simulink model "transmittingModel"  (R2024b)
settings: Solver=VariableStepAuto  StartTime=0.0  StopTime=inf  RelTol=1e-3
undefined symbols (not defined in the file or in its folder): designMultirateFIR, Fs, ip, j, usb
libraries: plutoradiolib x3, dspmlti4 x1, dspvision x1
settings Model: Creator=jldis  LastModifiedBy=jldis

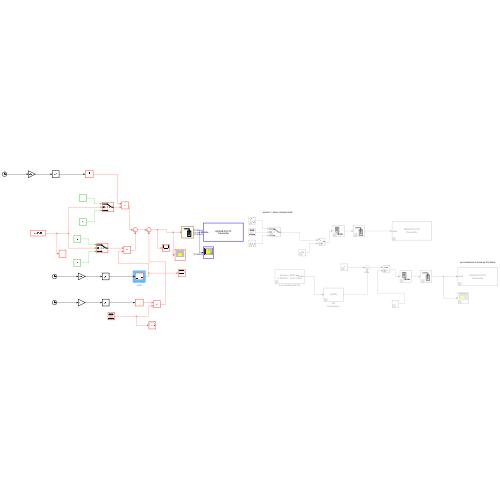
[thumbnail: Simulink's stored preview of the top-level diagram]
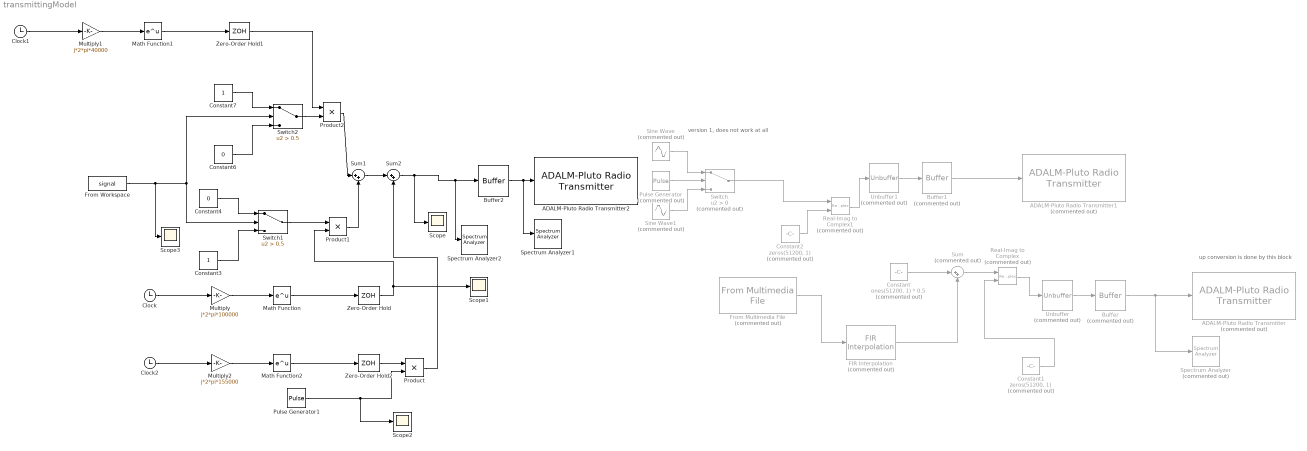
== system transmittingModel ==
  note: version 1, does not work at all
  note: up conversion is done by this block
  ADALM-Pluto Radio Transmitter : plutoradiolib/ADALM-Pluto Radio Transmitter  Commented=on  RadioID=usb:0  uri=ip:10.0.0.200  CenterFrequencySource=Dialog  CenterFrequency=915060000  GainSource=Dialog  Gain=-15  ChannelMapping=1  BasebandSampleRate=400000  UnderflowOutputPort=off  ShowAdvancedProperties=off  UseCustomFilter=off  filtPathRates=[737280000 11520000 3840000 1920000 960000 240000]  filtCoefficients=[-192 82 85 -215 228 -102 -110 290 -318 145 160 -426 471 -215 -238 633 -697 318 349 -923 1009 -457 -498 1309 -1423 640 693 -1812 1959 -876 -945 2458 -2647 1180 1268 -3290 3534 -1572 -1688 4375 -4698 2091 2247 -5836 6284 -2807 -3031 7918 -8588 3870 4225 -11182 12324 -5662 -6330 17255 -19735 9507 11312 -33568 43355 -25227 -42139 305542 305542 -42139 -25227 43355 -33568 11312 9507 -19735 17255 -6330 -5662 12324 -11182 4225 3870 -8588 7918 -3031 -2807 6284 -5836 2247 2091 -4698 4375 -1688 -1572 3534 -3290 1268 1180 -2647 2458 -945 -876 1959 -1812 693 640 -1423 1309 -498 -457 1009 -923 349 318 -697 633 -238 -215 471 -426 160 145 -318 290 -110 -102 228 -215 85 82 -192]  filtCoefficientSize=128  filtDecimInterpFactor=4  filtGain=-12  filtRFBandwidth=18000000  filterConfigStruct=struct()  DataSourceSelect=Input Port  DDSTone1Freq=5e3  DDSTone2Freq=10e3  DDSTone1Scale=0.5  DDSTone2Scale=0.25  DataTimeout=Inf  FrequencyCorrection=0  ENSMPinControlMode=None  BISTLoopbackMode=Disabled  BISTToneInject=Disabled  BISTSignalGen=PRBS  BISTToneFreq=Fs/32  BISTToneLevel=0
  ADALM-Pluto Radio Transmitter1 : plutoradiolib/ADALM-Pluto Radio Transmitter  Commented=on  RadioID=usb:0  uri=ip:10.0.0.200  CenterFrequencySource=Dialog  CenterFrequency=915060000  GainSource=Dialog  Gain=-15  ChannelMapping=1  BasebandSampleRate=400000  UnderflowOutputPort=off  ShowAdvancedProperties=off  UseCustomFilter=off  filtPathRates=[737280000 11520000 3840000 1920000 960000 240000]  filtCoefficients=[-192 82 85 -215 228 -102 -110 290 -318 145 160 -426 471 -215 -238 633 -697 318 349 -923 1009 -457 -498 1309 -1423 640 693 -1812 1959 -876 -945 2458 -2647 1180 1268 -3290 3534 -1572 -1688 4375 -4698 2091 2247 -5836 6284 -2807 -3031 7918 -8588 3870 4225 -11182 12324 -5662 -6330 17255 -19735 9507 11312 -33568 43355 -25227 -42139 305542 305542 -42139 -25227 43355 -33568 11312 9507 -19735 17255 -6330 -5662 12324 -11182 4225 3870 -8588 7918 -3031 -2807 6284 -5836 2247 2091 -4698 4375 -1688 -1572 3534 -3290 1268 1180 -2647 2458 -945 -876 1959 -1812 693 640 -1423 1309 -498 -457 1009 -923 349 318 -697 633 -238 -215 471 -426 160 145 -318 290 -110 -102 228 -215 85 82 -192]  filtCoefficientSize=128  filtDecimInterpFactor=4  filtGain=-12  filtRFBandwidth=18000000  filterConfigStruct=struct()  DataSourceSelect=Input Port  DDSTone1Freq=5e3  DDSTone2Freq=10e3  DDSTone1Scale=0.5  DDSTone2Scale=0.25  DataTimeout=Inf  FrequencyCorrection=0  ENSMPinControlMode=None  BISTLoopbackMode=Disabled  BISTToneInject=Disabled  BISTSignalGen=PRBS  BISTToneFreq=Fs/32  BISTToneLevel=0
  ADALM-Pluto Radio Transmitter2 : plutoradiolib/ADALM-Pluto Radio Transmitter  RadioID=usb:0  uri=ip:10.0.0.200  CenterFrequencySource=Dialog  CenterFrequency=913260000  GainSource=Dialog  Gain=-15  ChannelMapping=1  BasebandSampleRate=1000000  UnderflowOutputPort=off  ShowAdvancedProperties=off  UseCustomFilter=off  filtPathRates=[737280000 11520000 3840000 1920000 960000 240000]  filtCoefficients=[-192 82 85 -215 228 -102 -110 290 -318 145 160 -426 471 -215 -238 633 -697 318 349 -923 1009 -457 -498 1309 -1423 640 693 -1812 1959 -876 -945 2458 -2647 1180 1268 -3290 3534 -1572 -1688 4375 -4698 2091 2247 -5836 6284 -2807 -3031 7918 -8588 3870 4225 -11182 12324 -5662 -6330 17255 -19735 9507 11312 -33568 43355 -25227 -42139 305542 305542 -42139 -25227 43355 -33568 11312 9507 -19735 17255 -6330 -5662 12324 -11182 4225 3870 -8588 7918 -3031 -2807 6284 -5836 2247 2091 -4698 4375 -1688 -1572 3534 -3290 1268 1180 -2647 2458 -945 -876 1959 -1812 693 640 -1423 1309 -498 -457 1009 -923 349 318 -697 633 -238 -215 471 -426 160 145 -318 290 -110 -102 228 -215 85 82 -192]  filtCoefficientSize=128  filtDecimInterpFactor=4  filtGain=-12  filtRFBandwidth=18000000  filterConfigStruct=struct()  DataSourceSelect=Input Port  DDSTone1Freq=5e3  DDSTone2Freq=10e3  DDSTone1Scale=0.5  DDSTone2Scale=0.25  DataTimeout=Inf  FrequencyCorrection=0  ENSMPinControlMode=None  BISTLoopbackMode=Disabled  BISTToneInject=Disabled  BISTSignalGen=PRBS  BISTToneFreq=Fs/32  BISTToneLevel=0
  Buffer : Buffer  Commented=on  N=11226  OutputFrames=off
  Buffer1 : Buffer  Commented=on  N=11226  OutputFrames=off
  Buffer2 : Buffer  N=11226  OutputFrames=off
  Clock : Clock
      settings: Decimation=200000
  Clock1 : Clock
      settings: Decimation=200000
  Clock2 : Clock
      settings: Decimation=200000
  Constant : Constant  Commented=on  Value=ones(51200, 1) * 0.5  SampleTime=0.128
  Constant1 : Constant  Commented=on  Value=zeros(51200, 1)  SampleTime=0.128
  Constant2 : Constant  Commented=on  Value=zeros(51200, 1)  SampleTime=0.128
  Constant3 : Constant  SampleTime=1/1000000
  Constant4 : Constant  Value=0  SampleTime=1/1000000
  Constant6 : Constant  Value=0  SampleTime=1/1000000
  Constant7 : Constant  SampleTime=1/1000000
  FIR Interpolation : dspmlti4/FIR Interpolation  Commented=on  FilterSource=Auto  PrivateCoeffs=0  h=designMultirateFIR(3,1)  L=50  FilterObject=FINTERP  InputProcessing=Columns as channels (frame based)  framing=Enforce single-rate processing  outputBufInitCond=0  roundingMode=Floor  overflowMode=off  firstCoeffDataTypeStr=Inherit: Same word length as input  firstCoeffMin=[]  firstCoeffMax=[]  firstCoeffLastDataTypeStr=Inherit: Same word length as input  outputDataTypeStr=Inherit: Same as accumulator  outputMin=[]  outputMax=[]  outputLastDataTypeStr=Inherit: Same as accumulator
      settings: LibrarySourceBlock=|
      | dsphdlsupportfiltering/FIR
      | Interpolation
  From Workspace : FromWorkspace  VariableName=signal  SampleTime=.000001  Interpolate=off  OutputAfterFinalValue=Setting to zero
  From Multimedia File : dspvision/From Multimedia File  Commented=on  inputFilename=C:\Users\jldis\Downloads\blunders_8000.wav  readRange=[1 Inf]  loop=on  numPlays=inf  outputStreams=Audio only  videoDataType=single  audioDataType=double  inheritSampleTime=on  userDefinedSampleTime=1/30  noAudioOutput=off  isIntensityVideo=off  fourcc=RGB  colorVideoFormat=One multidimensional signal  outputEOF=off  dataOrg=Column-major  audioFrameSize=1024  computeAudioFrameSize=off  outSamplingMode=Sample based
      settings: LibrarySourceBlock=dspsrcs4/From Multimedia File
  Math Function : Math
  Math Function1 : Math
  Math Function2 : Math
  Multiply : Gain  Gain=j*2*pi*100000
  Multiply1 : Gain  Gain=j*2*pi*40000
  Multiply2 : Gain  Gain=j*2*pi*155000
  Product : Product
  Product1 : Product
  Product2 : Product
  Pulse Generator : DiscretePulseGenerator  Commented=on  Period=10  PulseWidth=10  SampleTime=1/4800
  Pulse Generator1 : DiscretePulseGenerator  Period=200000  PulseWidth=100000  SampleTime=1/1000000
  Real-Imag to Complex : RealImagToComplex  Commented=on
  Real-Imag to Complex1 : RealImagToComplex  Commented=on
  Scope{,1..3} (4 alike) : Scope
  Sine Wave : Sin  Commented=on  Frequency=915000000  SampleTime=1/1200
  Sine Wave1 : Sin  Commented=on  Frequency=915700000  SampleTime=1/1200
  Spectrum Analyzer : SpectrumAnalyzer  Commented=on  WindowPosition=[368.000000,182.000000,800.000000,500.000000,]  ScopeFrameLocation=window  WindowInvariantSamplesPerUpdate=on  Span=399999.99999999994  StartFrequency=-199999.99999999997  StopFrequency=199999.99999999997  YLimits=[-216.27025374,50.77893368]
  Spectrum Analyzer1 : SpectrumAnalyzer  WindowPosition=[-50.000000,181.000000,800.000000,500.000000,]  Visible=on  ScopeFrameLocation=window  WindowInvariantSamplesPerUpdate=on  Span=399999.99999999994  StartFrequency=-199999.99999999997  StopFrequency=199999.99999999997  YLimits=[-254.4855,61.60949983]
  Spectrum Analyzer2 : SpectrumAnalyzer  WindowPosition=[697.000000,189.000000,800.000000,500.000000,]  Visible=on  ScopeFrameLocation=window  WindowInvariantSamplesPerUpdate=on  Span=1000000  StartFrequency=-500000  StopFrequency=500000  YLimits=[-254.51263251,61.61251456]
  Sum : Sum  Commented=on  Inputs=|++
  Sum1 : Sum  Inputs=|++
  Sum2 : Sum  Inputs=|++
  Switch : Switch  Commented=on  Criteria=u2 > Threshold  SaturateOnIntegerOverflow=off  InputSameDT=off
  Switch1 : Switch  Criteria=u2 > Threshold  Threshold=0.5  SaturateOnIntegerOverflow=off  InputSameDT=off
  Switch2 : Switch  Criteria=u2 > Threshold  Threshold=0.5  SaturateOnIntegerOverflow=off  InputSameDT=off
  Unbuffer : Unbuffer  Commented=on
  Unbuffer1 : Unbuffer  Commented=on
  Zero-Order Hold : ZeroOrderHold  SampleTime=1/1000000
  Zero-Order Hold1 : ZeroOrderHold  SampleTime=1/1000000
  Zero-Order Hold2 : ZeroOrderHold  SampleTime=1/1000000
  wires:
  Buffer/1 -> Spectrum Analyzer/1, ADALM-Pluto Radio Transmitter/1
  Real-Imag to Complex/1 -> Unbuffer/1
  Unbuffer/1 -> Buffer/1
  Constant1/1 -> Real-Imag to Complex/2
  From Multimedia File/1 -> FIR Interpolation/1
  Sum/1 -> Real-Imag to Complex/1
  Constant/1 -> Sum/1
  FIR Interpolation/1 -> Sum/2
  Pulse Generator/1 -> Switch/2
  Sine Wave1/1 -> Switch/3
  Sine Wave/1 -> Switch/1
  Buffer1/1 -> ADALM-Pluto Radio Transmitter1/1
  Unbuffer1/1 -> Buffer1/1
  Switch/1 -> Real-Imag to Complex1/1
  Constant2/1 -> Real-Imag to Complex1/2
  Real-Imag to Complex1/1 -> Unbuffer1/1
  Constant3/1 -> Switch1/3
  Constant4/1 -> Switch1/1
  Switch1/1 -> Product1/1
  Product1/1 -> Sum1/2
  Multiply/1 -> Math Function/1
  Clock/1 -> Multiply/1
  Math Function/1 -> Zero-Order Hold/1
  Constant7/1 -> Switch2/1
  Constant6/1 -> Switch2/3
  Math Function1/1 -> Zero-Order Hold1/1
  Zero-Order Hold1/1 -> Product2/1
  Multiply1/1 -> Math Function1/1
  Clock1/1 -> Multiply1/1
  Product2/1 -> Sum1/1
  Switch2/1 -> Product2/2
  From Workspace/1 -> Scope3/1, Switch1/2, Switch2/2
  Zero-Order Hold/1 -> Scope1/1, Product1/2
  Clock2/1 -> Multiply2/1
  Multiply2/1 -> Math Function2/1
  Math Function2/1 -> Zero-Order Hold2/1
  Zero-Order Hold2/1 -> Product/1
  Pulse Generator1/1 -> Scope2/1, Product/2
  Buffer2/1 -> Spectrum Analyzer1/1, ADALM-Pluto Radio Transmitter2/1
  Sum1/1 -> Sum2/1
  Product/1 -> Sum2/2
  Sum2/1 -> Spectrum Analyzer2/1, Buffer2/1, Scope/1
